simulink model "fuzzy_controller"  (R2021a)
settings: Solver=VariableStepAuto  StartTime=0.0  StopTime=20  RelTol=1e-3
libraries: fuzblock x1
settings Model: Creator=User  LastModifiedBy=User

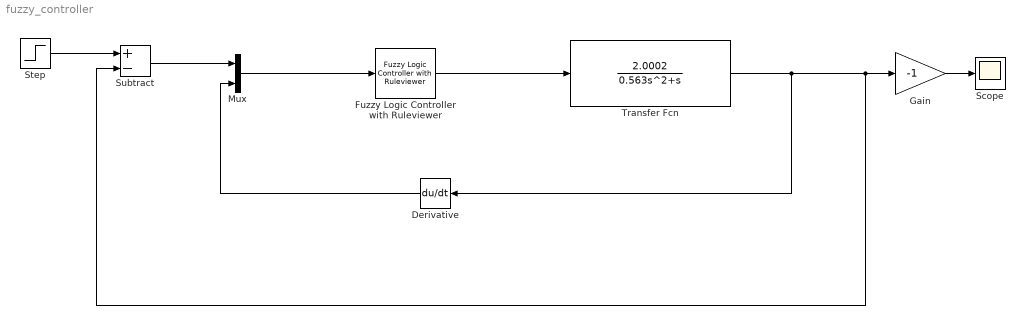
== system fuzzy_controller ==
  Derivative : Derivative
  Fuzzy Logic Controller with Ruleviewer : fuzblock/Fuzzy Logic  Controller  with Ruleviewer  fismatrix=rules  Ts=2
  Gain : Gain  Gain=-1
  Mux : Mux  Inputs=2
  Scope : Scope
  Step : Step  Time=0  After=10  SampleTime=0
  Subtract : Sum  Inputs=+-
  Transfer Fcn : TransferFcn  Numerator=[2.0002]  Denominator=[0.563 1 0]
  wires:
  Step/1 -> Subtract/1
  Subtract/1 -> Mux/1
  Mux/1 -> Fuzzy Logic Controller with Ruleviewer/1
  Fuzzy Logic Controller with Ruleviewer/1 -> Transfer Fcn/1
  Derivative/1 -> Mux/2
  Transfer Fcn/1 -> Derivative/1, Subtract/2, Gain/1
  Gain/1 -> Scope/1
